simulink model "PenduloInvKalmanFunc"  (R2019b)
settings: Solver=VariableStepAuto  StartTime=0.0  StopTime=15  RelTol=1e-3
libraries: simulink x1, sharedTrackingLibrary x1
settings Model: Creator=Guzo  LastModifiedBy=Guzo

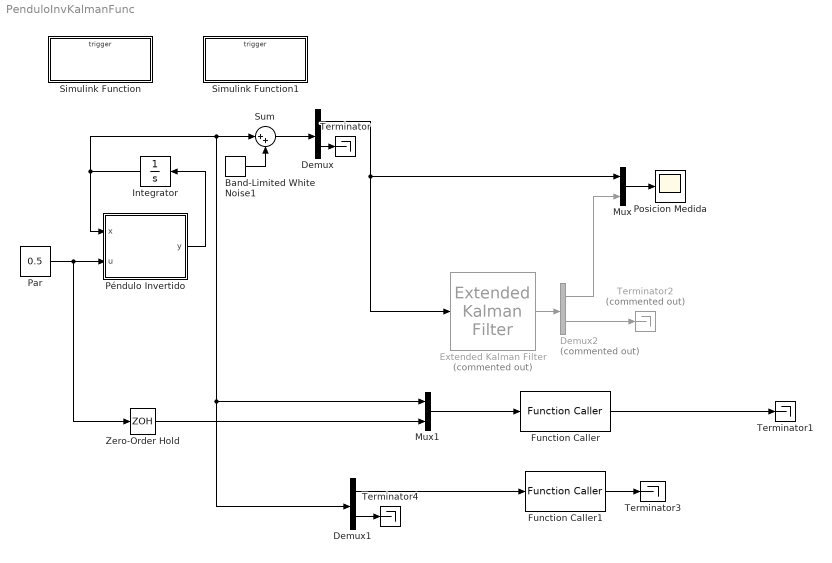
== system PenduloInvKalmanFunc ==
  Band-Limited White Noise1 : simulink/Sources/Band-Limited White Noise  Cov=1e-5*0.1  Ts=0.01  seed=[23942]
  Demux : Demux  Outputs=2
  Demux1 : Demux  Outputs=2
  Demux2 : Demux  Commented=on  Outputs=2
  Extended Kalman Filter : sharedTrackingLibrary/Extended Kalman Filter  Commented=on  StateTransitionFcn=PenduloInv  HasStateTransitionJacobianFcn=off  HasAdditiveProcessNoise=Additive  ProcessNoise=diag([0 1e-3])  HasTimeVaryingProcessNoise=off  HasStateTransitionFcnExtraArgument=0  InitialState=[0 0]  InitialStateCovariance=1e-3  MeasurementFcn1=Medida  HasMeasurementJacobianFcn1=off  HasMeasurementEnablePort1=off  HasAdditiveMeasurementNoise1=Additive  MeasurementNoise1=1e-5  HasTimeVaryingMeasurementNoise1=off  HasMeasurementFcnExtraArgument1=0  MeasurementFcn2=myMeasurementFcn  HasMeasurementJacobianFcn2=off  HasMeasurementEnablePort2=off  HasAdditiveMeasurementNoise2=Additive  MeasurementNoise2=1  HasTimeVaryingMeasurementNoise2=off  HasMeasurementFcnExtraArgument2=0  MeasurementFcn3=myMeasurementFcn  HasMeasurementJacobianFcn3=off  HasMeasurementEnablePort3=off  HasAdditiveMeasurementNoise3=Additive  MeasurementNoise3=1  HasTimeVaryingMeasurementNoise3=off  HasMeasurementFcnExtraArgument3=0  MeasurementFcn4=myMeasurementFcn  HasMeasurementJacobianFcn4=off  HasMeasurementEnablePort4=off  HasAdditiveMeasurementNoise4=Additive  MeasurementNoise4=1  HasTimeVaryingMeasurementNoise4=off  HasMeasurementFcnExtraArgument4=0  MeasurementFcn5=myMeasurementFcn  HasMeasurementJacobianFcn5=off  HasMeasurementEnablePort5=off  HasAdditiveMeasurementNoise5=Additive  MeasurementNoise5=1  HasTimeVaryingMeasurementNoise5=off  HasMeasurementFcnExtraArgument5=0  EnableMultirate=off  StateTransitionFcnSampleTime=1  MeasurementFcn1SampleTime=1  MeasurementFcn2SampleTime=1  MeasurementFcn3SampleTime=1  MeasurementFcn4SampleTime=1  MeasurementFcn5SampleTime=1  UseCurrentEstimator=on  OutputStateCovariance=off  DataType=double  SampleTime=0.02  NumberOfMeasurements=1
      settings: SourceProductName=Automated Driving Toolbox  SourceProductBaseCode=DR
  Function Caller : FunctionCaller  FunctionPrototype=x = PenduloInv(u)  InputArgumentSpecifications=[1,3]  OutputArgumentSpecifications=[1,3]
  Function Caller1 : FunctionCaller  FunctionPrototype=x = Medida(x)  InputArgumentSpecifications=1  OutputArgumentSpecifications=1
  Integrator : Integrator  InitialCondition=[0;0]
  Mux : Mux  Inputs=2
  Mux1 : Mux  Inputs=2
  Par : Constant  Value=0.5
  Posicion Medida : Scope
  Péndulo Invertido : MATLAB Function  TreatAsAtomicUnit=on
  Simulink Function : Subsystem  TreatAsAtomicUnit=on
  Simulink Function1 : Subsystem  TreatAsAtomicUnit=on
  Sum : Sum  Inputs=|++
  Terminator{,1,3..4} (4 alike) : Terminator
  Terminator2 : Terminator  Commented=on
  Zero-Order Hold : ZeroOrderHold  SampleTime=0.02
  wires:
  Péndulo Invertido/1(y) -> Integrator/1
  Par/1 -> Péndulo Invertido/2(u), Zero-Order Hold/1
  Sum/1 -> Demux/1
  Demux/2 -> Terminator/1
  Band-Limited White Noise1/1 -> Sum/2
  Mux/1 -> Posicion Medida/1
  Demux2/2 -> Terminator2/1
  Extended Kalman Filter/1 -> Demux2/1
  Demux/1 -> Extended Kalman Filter/1, Mux/1
  Demux2/1 -> Mux/2
  Function Caller/1 -> Terminator1/1
  Function Caller1/1 -> Terminator3/1
  Integrator/1 -> Sum/1, Mux1/1, Demux1/1, Péndulo Invertido/1(x)
  Demux1/1 -> Function Caller1/1
  Demux1/2 -> Terminator4/1
  Mux1/1 -> Function Caller/1
  Zero-Order Hold/1 -> Mux1/2

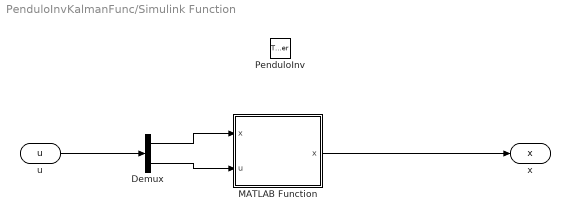
== system PenduloInvKalmanFunc/Simulink Function ==
  PenduloInv : TriggerPort  TriggerType=function-call  IsSimulinkFunction=on  FunctionName=PenduloInv  Variant=on  VariantControl=(inherit)
  Demux : Demux  Outputs=2
  MATLAB Function : MATLAB Function  TreatAsAtomicUnit=on
  u : ArgIn  DisableCoverage=on  PortDimensions=[1,3]  ArgumentName=u
  x : ArgOut  DisableCoverage=on  PortDimensions=[1,2]  ArgumentName=x
  wires:
  MATLAB Function/1(x) -> x/1
  u/1 -> Demux/1
  Demux/1 -> MATLAB Function/1("x ")
  Demux/2 -> MATLAB Function/2(u)

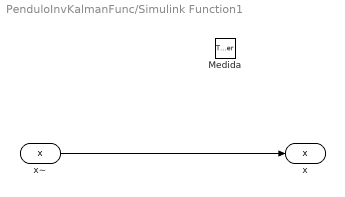
== system PenduloInvKalmanFunc/Simulink Function1 ==
  Medida : TriggerPort  TriggerType=function-call  IsSimulinkFunction=on  FunctionName=Medida  FunctionVisibility=scoped  VariantControl=(inherit)
  x~ : ArgIn  DisableCoverage=on  ArgumentName=x
  x : ArgOut  DisableCoverage=on  ArgumentName=x
  wires:
  x~/1 -> x/1

== matlab function PenduloInvKalmanFunc/Simulink Function/MATLAB Function ==
  data: x input; u input; x output
function x = PenduloInv(x,u)
%Constantes del sistema
g=9.81;
l=1;
m=0.75;
b=0.5;

%Tiempo de muestreo
t = 0.01;

x = x+[x(2);(g/l)*sin(x(1))-(b/(m*l^2))*x(2)+(1/(m*l^2))*u]*t;

end

== matlab function PenduloInvKalmanFunc/Péndulo Invertido ==
  data: x input; y output; u input
function y  = fcn(x,u)
g=9.81;
l=1;
m=0.75;
b=0.5;

x1 = x(1);
x2 = x(2);

xp=[x2;(g/l)*sin(x1)-(b/(m*l^2))*x2+(1/(m*l^2))*u];

y = xp;
